simulink model "CounterUp"  (R2016a)
settings: Solver=FixedStepDiscrete  StartTime=0.0  StopTime=10.0  RelTol=1e-3
model workspace (MAT data in the model file):
  cs : Simulink.ConfigSet (value not decoded)
settings Model: Creator=LEGION  LastModifiedBy=LEGION

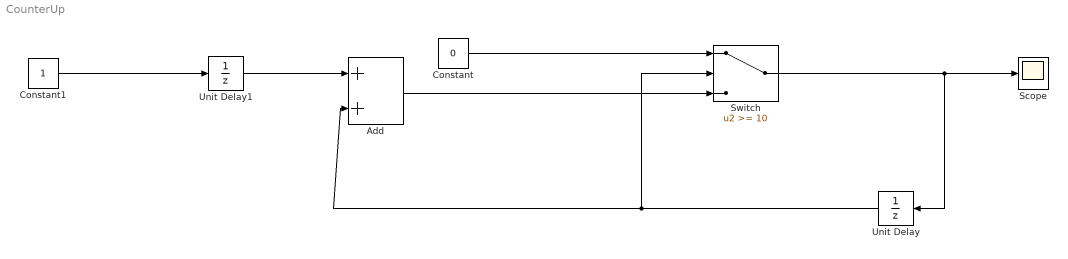
== system CounterUp ==
  Add : Sum
  Constant : Constant  Value=0
  Constant1 : Constant
  Scope : Scope
  Switch : Switch  Threshold=10
  Unit Delay : UnitDelay  SampleTime=-1
  Unit Delay1 : UnitDelay  SampleTime=-1
  wires:
  Switch/1 -> Unit Delay/1, Scope/1
  Unit Delay/1 -> Switch/2, Add/2
  Add/1 -> Switch/3
  Constant/1 -> Switch/1
  Constant1/1 -> Unit Delay1/1
  Unit Delay1/1 -> Add/1
